simulink model "Dead_Space_Khoo"  (Simulink 6.4)
settings: Solver=ode45  StartTime=0.0  StopTime=10.0  RelTol=1e-3
values from neighbouring files (symbols this model uses):
  Dead1CO2IC = 0.1020    (= 0.102)    [Dead_Space_Khoo_IC.m]    (also in Gas_Exchange_IC.m; Respiratory_IC.m = 39.5616)
  Dead1O2IC = 149.8824    [Dead_Space_Khoo_IC.m]    (also in Gas_Exchange_IC.m; Respiratory_IC.m = 104.3637)
  Dead2CO2IC = 0.5274    [Dead_Space_Khoo_IC.m]    (also in Gas_Exchange_IC.m; Respiratory_IC.m = 39.6736)
  Dead2O2IC = 149.3923    [Dead_Space_Khoo_IC.m]    (also in Gas_Exchange_IC.m; Respiratory_IC.m = 104.2258)
  Dead3CO2IC = 2.2996    [Dead_Space_Khoo_IC.m]    (also in Gas_Exchange_IC.m; Respiratory_IC.m = 39.8127)
  Dead3O2IC = 147.3503    [Dead_Space_Khoo_IC.m]    (also in Gas_Exchange_IC.m; Respiratory_IC.m = 104.0505)
  Dead4CO2IC = 8.2293    [Dead_Space_Khoo_IC.m]    (also in Gas_Exchange_IC.m; Respiratory_IC.m = 40.0061)
  Dead4O2IC = 140.5179    [Dead_Space_Khoo_IC.m]    (also in Gas_Exchange_IC.m; Respiratory_IC.m = 103.8005)
  Dead5CO2IC = 22.0757    [Dead_Space_Khoo_IC.m]    (also in Gas_Exchange_IC.m; Respiratory_IC.m = 40.3359)
  Dead5O2IC = 124.5641    [Dead_Space_Khoo_IC.m]    (also in Gas_Exchange_IC.m; Respiratory_IC.m = 103.3579)
  PICO2 = 0    [Dead_Space_Khoo_IC.m]    (also in Gas_Exchange_IC.m; Respiratory_IC.m)
  PICO2_change = 0    [Respiratory_IC.m]
  PIO2 = 150    [Dead_Space_Khoo_IC.m]    (also in Gas_Exchange_IC.m; Respiratory_IC.m)
  PIO2_change = -90    [Mech_vent_test.m]    (also in Respiratory_IC.m = 0)
  t_CO2_duration = 0    [Respiratory_IC.m]
  t_CO2_start = 0    [Respiratory_IC.m]
  t_O2_duration = 0    [Mech_vent_test.m]    (also in Respiratory_IC.m)
  t_O2_start = 0    [Mech_vent_test.m]    (also in Respiratory_IC.m)
  Vdead1 = 0.03    [Dead_Space_Khoo_IC.m]    (also in Gas_Exchange_IC.m; Respiratory_IC.m)
  Vdead2 = 0.03    [Dead_Space_Khoo_IC.m]    (also in Gas_Exchange_IC.m; Respiratory_IC.m)
  Vdead3 = 0.03    [Dead_Space_Khoo_IC.m]    (also in Gas_Exchange_IC.m; Respiratory_IC.m)
  Vdead4 = 0.03    [Dead_Space_Khoo_IC.m]    (also in Gas_Exchange_IC.m; Respiratory_IC.m)
  Vdead5 = 0.03    [Dead_Space_Khoo_IC.m]    (also in Gas_Exchange_IC.m; Respiratory_IC.m)
settings Model: LastModifiedBy=CLM
settings OptimizationCC: BlockReduction=off  BooleanDataType=off
settings DebuggingCC: SolverPrmCheckMsg=none  StrictBusMsg=None
settings HardwareCC: TargetUnknown=on

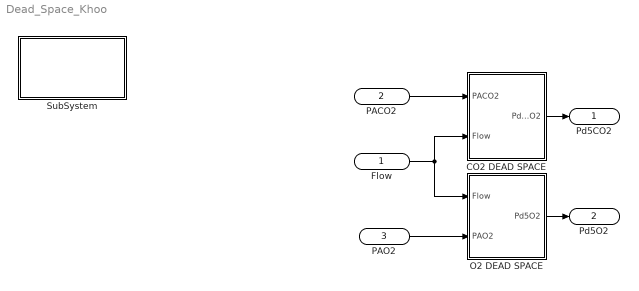
== system Dead_Space_Khoo ==
  Flow : Inport
  PACO2 : Inport  Port=2
  PAO2 : Inport  Port=3
  CO2 DEAD SPACE : Subsystem
  O2 DEAD SPACE : Subsystem
  SubSystem : Subsystem
      settings: OpenFcn=Baro_Ursino_IC
      mask Display: disp('"double click here"\n to load \nDead_Space_Khoo \ninitial values');
  Pd5CO2 : Outport
  Pd5O2 : Outport  Port=2
  wires:
  Flow/1 -> CO2 DEAD SPACE/2(Flow), O2 DEAD SPACE/1(Flow)
  O2 DEAD SPACE/1(Pd5O2) -> Pd5O2/1
  CO2 DEAD SPACE/1(Pd5CO2) -> Pd5CO2/1
  PAO2/1 -> O2 DEAD SPACE/2(PAO2)
  PACO2/1 -> CO2 DEAD SPACE/1(PACO2)

== system Dead_Space_Khoo/CO2 DEAD SPACE ==
  PACO2 : Inport
  Flow : Inport  Port=2
  CO2 Partial Pressure : Subsystem  mask{begin_time=t_CO2_start, end_time=t_CO2_start+t_CO2_duration, init_value=PICO2, final_value=PICO2+PICO2_change}
      mask prompts: begin_time "pulse begin"; end_time "pulse end"; init_value "initial value"; final_value "final value"
      mask Display: disp('pulse')
  Pd(1)CO2 : Subsystem
  Pd(2)CO2 : Subsystem
  Pd(3)CO2 : Subsystem
  Pd(4)CO2 : Subsystem
  Pd(5)CO2 : Subsystem
  Pd5CO2 : Outport
  wires:
  Pd(4)CO2/1(Pd(4)CO2) -> Pd(3)CO2/3(Pd(4)CO2), Pd(5)CO2/1(Pd(4)CO2)
  Pd(3)CO2/1(Pd(3)CO2) -> Pd(2)CO2/3(Pd(3)CO2), Pd(4)CO2/1(Pd(3)CO2)
  Pd(2)CO2/1(Pd(2)CO2) -> Pd(1)CO2/3(Pd(2)CO2), Pd(3)CO2/1(Pd(2)CO2)
  Pd(1)CO2/1(Pd(1)CO2) -> Pd(2)CO2/1(Pd(1)CO2)
  Flow/1 -> Pd(1)CO2/2(Flow), Pd(2)CO2/2(Flow), Pd(5)CO2/2(Flow), Pd(4)CO2/2(Flow), Pd(3)CO2/2(Flow)
  PACO2/1 -> Pd(5)CO2/3(PACO2)
  Pd(5)CO2/1(Pd(5)CO2) -> Pd5CO2/1, Pd(4)CO2/3(Pd(5)CO2)
  CO2 Partial Pressure/1(Out1) -> Pd(1)CO2/1(PICO2)

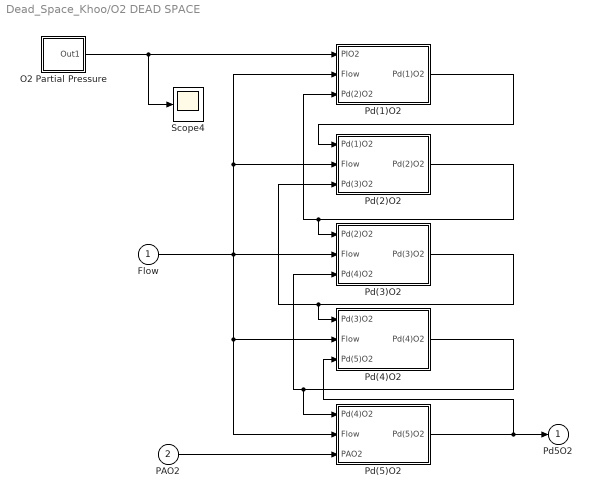
== system Dead_Space_Khoo/O2 DEAD SPACE ==
  Flow : Inport
  PAO2 : Inport  Port=2
  O2 Partial Pressure : Subsystem  mask{begin_time=t_O2_start, end_time=t_O2_start+t_O2_duration, init_value=PIO2, final_value=PIO2+PIO2_change}
      mask prompts: begin_time "pulse begin"; end_time "pulse end"; init_value "initial value"; final_value "final value"
      mask Display: disp('pulse')
  Pd(1)O2 : Subsystem
  Pd(2)O2 : Subsystem
  Pd(3)O2 : Subsystem
  Pd(4)O2 : Subsystem
  Pd(5)O2 : Subsystem
  Scope4 : Scope
      settings: YMin=97.7  YMax=98.3  SaveName=ScopeData40
  Pd5O2 : Outport
  wires:
  Pd(4)O2/1(Pd(4)O2) -> Pd(5)O2/1(Pd(4)O2), Pd(3)O2/3(Pd(4)O2)
  Pd(3)O2/1(Pd(3)O2) -> Pd(2)O2/3(Pd(3)O2), Pd(4)O2/1(Pd(3)O2)
  Pd(2)O2/1(Pd(2)O2) -> Pd(1)O2/3(Pd(2)O2), Pd(3)O2/1(Pd(2)O2)
  Pd(1)O2/1(Pd(1)O2) -> Pd(2)O2/1(Pd(1)O2)
  PAO2/1 -> Pd(5)O2/3(PAO2)
  Flow/1 -> Pd(5)O2/2(Flow), Pd(4)O2/2(Flow), Pd(1)O2/2(Flow), Pd(2)O2/2(Flow), Pd(3)O2/2(Flow)
  Pd(5)O2/1(Pd(5)O2) -> Pd5O2/1, Pd(4)O2/3(Pd(5)O2)
  O2 Partial Pressure/1(Out1) -> Pd(1)O2/1(PIO2), Scope4/1

== system Dead_Space_Khoo/SubSystem ==

== system Dead_Space_Khoo/CO2 DEAD SPACE/CO2 Partial Pressure ==
  Step : Step  Time=begin_time  Before=init_value  After=final_value  SampleTime=0
  Step1 : Step  Time=end_time  After=init_value-final_value  SampleTime=0
  Sum : Sum  Inputs=|++  SaturateOnIntegerOverflow=on  InputSameDT=on
  Out1 : Outport
  wires:
  Step/1 -> Sum/1
  Step1/1 -> Sum/2
  Sum/1 -> Out1/1

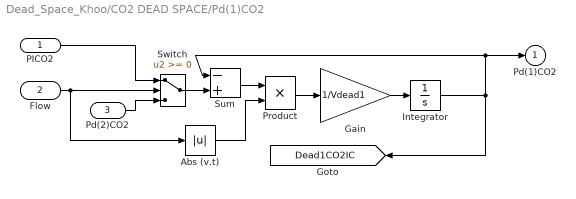
== system Dead_Space_Khoo/CO2 DEAD SPACE/Pd(1)CO2 ==
  PICO2 : Inport
  Flow : Inport  Port=2
  Pd(2)CO2 : Inport  Port=3
  Abs (v.t) : Abs  SaturateOnIntegerOverflow=on  SampleTime=-1
  Gain : Gain  Gain=1/Vdead1  SaturateOnIntegerOverflow=on
  Integrator : Integrator  InitialCondition=Dead1CO2IC
  Product : Product  SaturateOnIntegerOverflow=on  RndMeth=Zero  InputSameDT=on
  Sum : Sum  Inputs=-+  SaturateOnIntegerOverflow=on  InputSameDT=on
  Switch : Switch  SaturateOnIntegerOverflow=on  InputSameDT=on
  Pd(1)CO2 : Outport
  tag scope: Dead1CO2IC=global
  wires:
  Flow/1 -> Abs (v.t)/1, Switch/2
  Abs (v.t)/1 -> Product/2
  Switch/1 -> Sum/2
  Product/1 -> Gain/1
  Gain/1 -> Integrator/1
  Integrator/1 -> Sum/1, Pd(1)CO2/1, [Dead1CO2IC]
  Sum/1 -> Product/1
  PICO2/1 -> Switch/1
  Pd(2)CO2/1 -> Switch/3

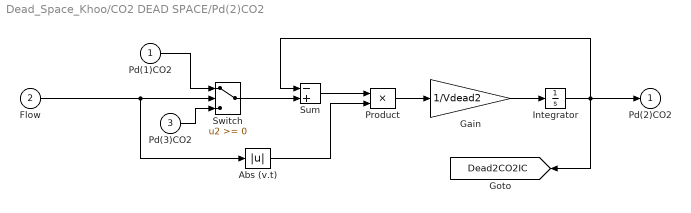
== system Dead_Space_Khoo/CO2 DEAD SPACE/Pd(2)CO2 ==
  Pd(1)CO2 : Inport
  Flow : Inport  Port=2
  Pd(3)CO2 : Inport  Port=3
  Abs (v.t) : Abs  SaturateOnIntegerOverflow=on  SampleTime=-1
  Gain : Gain  Gain=1/Vdead2  SaturateOnIntegerOverflow=on
  Integrator : Integrator  InitialCondition=Dead2CO2IC
  Product : Product  SaturateOnIntegerOverflow=on  RndMeth=Zero  InputSameDT=on
  Sum : Sum  Inputs=-+  SaturateOnIntegerOverflow=on  InputSameDT=on
  Switch : Switch  SaturateOnIntegerOverflow=on  InputSameDT=on
  Pd(2)CO2 : Outport
  tag scope: Dead2CO2IC=global
  wires:
  Integrator/1 -> Sum/1, Pd(2)CO2/1, [Dead2CO2IC]
  Abs (v.t)/1 -> Product/2
  Flow/1 -> Abs (v.t)/1, Switch/2
  Pd(3)CO2/1 -> Switch/3
  Pd(1)CO2/1 -> Switch/1
  Sum/1 -> Product/1
  Gain/1 -> Integrator/1
  Product/1 -> Gain/1
  Switch/1 -> Sum/2

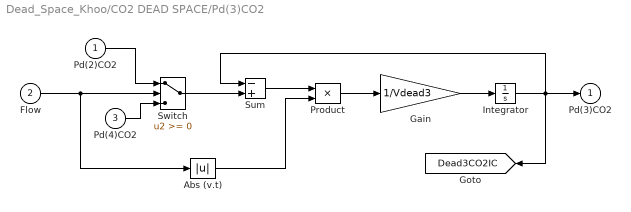
== system Dead_Space_Khoo/CO2 DEAD SPACE/Pd(3)CO2 ==
  Pd(2)CO2 : Inport
  Flow : Inport  Port=2
  Pd(4)CO2 : Inport  Port=3
  Abs (v.t) : Abs  SaturateOnIntegerOverflow=on  SampleTime=-1
  Gain : Gain  Gain=1/Vdead3  SaturateOnIntegerOverflow=on
  Integrator : Integrator  InitialCondition=Dead3CO2IC
  Product : Product  SaturateOnIntegerOverflow=on  RndMeth=Zero  InputSameDT=on
  Sum : Sum  Inputs=-+  SaturateOnIntegerOverflow=on  InputSameDT=on
  Switch : Switch  SaturateOnIntegerOverflow=on  InputSameDT=on
  Pd(3)CO2 : Outport
  tag scope: Dead3CO2IC=global
  wires:
  Abs (v.t)/1 -> Product/2
  Flow/1 -> Abs (v.t)/1, Switch/2
  Switch/1 -> Sum/2
  Product/1 -> Gain/1
  Gain/1 -> Integrator/1
  Integrator/1 -> Sum/1, Pd(3)CO2/1, [Dead3CO2IC]
  Sum/1 -> Product/1
  Pd(2)CO2/1 -> Switch/1
  Pd(4)CO2/1 -> Switch/3

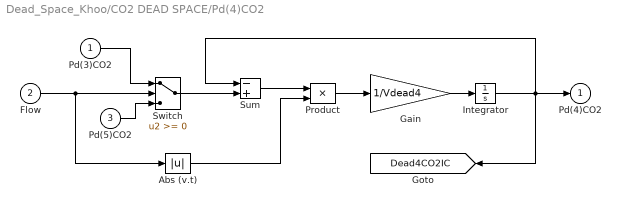
== system Dead_Space_Khoo/CO2 DEAD SPACE/Pd(4)CO2 ==
  Pd(3)CO2 : Inport
  Flow : Inport  Port=2
  Pd(5)CO2 : Inport  Port=3
  Abs (v.t) : Abs  SaturateOnIntegerOverflow=on  SampleTime=-1
  Gain : Gain  Gain=1/Vdead4  SaturateOnIntegerOverflow=on
  Integrator : Integrator  InitialCondition=Dead4CO2IC
  Product : Product  SaturateOnIntegerOverflow=on  RndMeth=Zero  InputSameDT=on
  Sum : Sum  Inputs=-+  SaturateOnIntegerOverflow=on  InputSameDT=on
  Switch : Switch  SaturateOnIntegerOverflow=on  InputSameDT=on
  Pd(4)CO2 : Outport
  tag scope: Dead4CO2IC=global
  wires:
  Integrator/1 -> Sum/1, Pd(4)CO2/1, [Dead4CO2IC]
  Abs (v.t)/1 -> Product/2
  Flow/1 -> Abs (v.t)/1, Switch/2
  Pd(5)CO2/1 -> Switch/3
  Pd(3)CO2/1 -> Switch/1
  Sum/1 -> Product/1
  Gain/1 -> Integrator/1
  Product/1 -> Gain/1
  Switch/1 -> Sum/2

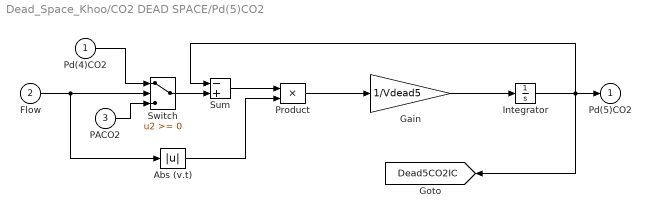
== system Dead_Space_Khoo/CO2 DEAD SPACE/Pd(5)CO2 ==
  Pd(4)CO2 : Inport
  Flow : Inport  Port=2
  PACO2 : Inport  Port=3
  Abs (v.t) : Abs  SaturateOnIntegerOverflow=on  SampleTime=-1
  Gain : Gain  Gain=1/Vdead5  SaturateOnIntegerOverflow=on
  Integrator : Integrator  InitialCondition=Dead5CO2IC
  Product : Product  SaturateOnIntegerOverflow=on  RndMeth=Zero  InputSameDT=on
  Sum : Sum  Inputs=-+  SaturateOnIntegerOverflow=on  InputSameDT=on
  Switch : Switch  SaturateOnIntegerOverflow=on  InputSameDT=on
  Pd(5)CO2 : Outport
  tag scope: Dead5CO2IC=global
  wires:
  Abs (v.t)/1 -> Product/2
  Flow/1 -> Abs (v.t)/1, Switch/2
  Switch/1 -> Sum/2
  Product/1 -> Gain/1
  Gain/1 -> Integrator/1
  Integrator/1 -> Sum/1, Pd(5)CO2/1, [Dead5CO2IC]
  Sum/1 -> Product/1
  Pd(4)CO2/1 -> Switch/1
  PACO2/1 -> Switch/3

== system Dead_Space_Khoo/O2 DEAD SPACE/O2 Partial Pressure ==
  Step : Step  Time=begin_time  Before=init_value  After=final_value  SampleTime=0
  Step1 : Step  Time=end_time  After=init_value-final_value  SampleTime=0
  Sum : Sum  Inputs=|++  SaturateOnIntegerOverflow=on  InputSameDT=on
  Out1 : Outport
  wires:
  Sum/1 -> Out1/1
  Step1/1 -> Sum/2
  Step/1 -> Sum/1

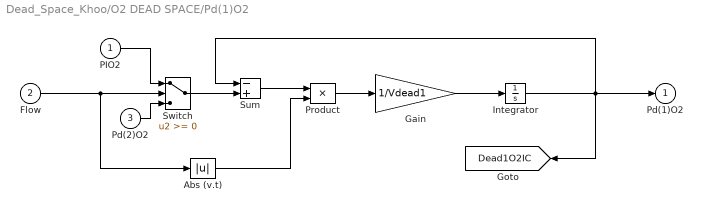
== system Dead_Space_Khoo/O2 DEAD SPACE/Pd(1)O2 ==
  PIO2 : Inport
  Flow : Inport  Port=2
  Pd(2)O2 : Inport  Port=3
  Abs (v.t) : Abs  SaturateOnIntegerOverflow=on  SampleTime=-1
  Gain : Gain  Gain=1/Vdead1  SaturateOnIntegerOverflow=on
  Integrator : Integrator  InitialCondition=Dead1O2IC
  Product : Product  SaturateOnIntegerOverflow=on  RndMeth=Zero  InputSameDT=on
  Sum : Sum  Inputs=-+  SaturateOnIntegerOverflow=on  InputSameDT=on
  Switch : Switch  SaturateOnIntegerOverflow=on  InputSameDT=on
  Pd(1)O2 : Outport
  tag scope: Dead1O2IC=global
  wires:
  Switch/1 -> Sum/2
  Pd(2)O2/1 -> Switch/3
  PIO2/1 -> Switch/1
  Sum/1 -> Product/1
  Integrator/1 -> Sum/1, Pd(1)O2/1, [Dead1O2IC]
  Gain/1 -> Integrator/1
  Product/1 -> Gain/1
  Flow/1 -> Abs (v.t)/1, Switch/2
  Abs (v.t)/1 -> Product/2

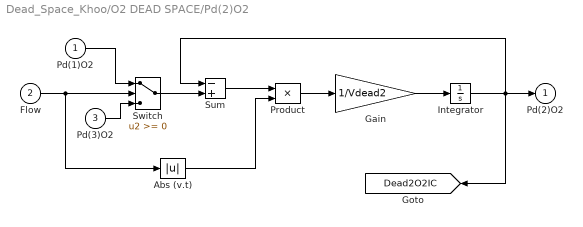
== system Dead_Space_Khoo/O2 DEAD SPACE/Pd(2)O2 ==
  Pd(1)O2 : Inport
  Flow : Inport  Port=2
  Pd(3)O2 : Inport  Port=3
  Abs (v.t) : Abs  SaturateOnIntegerOverflow=on  SampleTime=-1
  Gain : Gain  Gain=1/Vdead2  SaturateOnIntegerOverflow=on
  Integrator : Integrator  InitialCondition=Dead2O2IC
  Product : Product  SaturateOnIntegerOverflow=on  RndMeth=Zero  InputSameDT=on
  Sum : Sum  Inputs=-+  SaturateOnIntegerOverflow=on  InputSameDT=on
  Switch : Switch  SaturateOnIntegerOverflow=on  InputSameDT=on
  Pd(2)O2 : Outport
  tag scope: Dead2O2IC=global
  wires:
  Abs (v.t)/1 -> Product/2
  Flow/1 -> Abs (v.t)/1, Switch/2
  Product/1 -> Gain/1
  Integrator/1 -> [Dead2O2IC], Sum/1, Pd(2)O2/1
  Sum/1 -> Product/1
  Pd(1)O2/1 -> Switch/1
  Pd(3)O2/1 -> Switch/3
  Switch/1 -> Sum/2
  Gain/1 -> Integrator/1

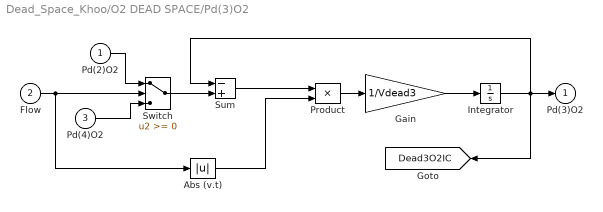
== system Dead_Space_Khoo/O2 DEAD SPACE/Pd(3)O2 ==
  Pd(2)O2 : Inport
  Flow : Inport  Port=2
  Pd(4)O2 : Inport  Port=3
  Abs (v.t) : Abs  SaturateOnIntegerOverflow=on  SampleTime=-1
  Gain : Gain  Gain=1/Vdead3  SaturateOnIntegerOverflow=on
  Integrator : Integrator  InitialCondition=Dead3O2IC
  Product : Product  SaturateOnIntegerOverflow=on  RndMeth=Zero  InputSameDT=on
  Sum : Sum  Inputs=-+  SaturateOnIntegerOverflow=on  InputSameDT=on
  Switch : Switch  SaturateOnIntegerOverflow=on  InputSameDT=on
  Pd(3)O2 : Outport
  tag scope: Dead3O2IC=global
  wires:
  Switch/1 -> Sum/2
  Pd(4)O2/1 -> Switch/3
  Pd(2)O2/1 -> Switch/1
  Sum/1 -> Product/1
  Integrator/1 -> [Dead3O2IC], Sum/1, Pd(3)O2/1
  Product/1 -> Gain/1
  Flow/1 -> Abs (v.t)/1, Switch/2
  Abs (v.t)/1 -> Product/2
  Gain/1 -> Integrator/1

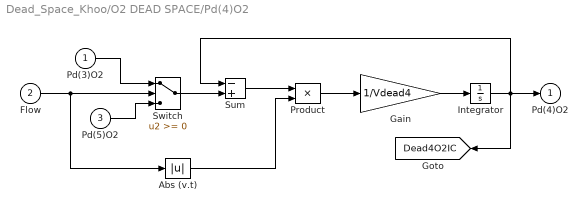
== system Dead_Space_Khoo/O2 DEAD SPACE/Pd(4)O2 ==
  Pd(3)O2 : Inport
  Flow : Inport  Port=2
  Pd(5)O2 : Inport  Port=3
  Abs (v.t) : Abs  SaturateOnIntegerOverflow=on  SampleTime=-1
  Gain : Gain  Gain=1/Vdead4  SaturateOnIntegerOverflow=on
  Integrator : Integrator  InitialCondition=Dead4O2IC
  Product : Product  SaturateOnIntegerOverflow=on  RndMeth=Zero  InputSameDT=on
  Sum : Sum  Inputs=-+  SaturateOnIntegerOverflow=on  InputSameDT=on
  Switch : Switch  SaturateOnIntegerOverflow=on  InputSameDT=on
  Pd(4)O2 : Outport
  tag scope: Dead4O2IC=global
  wires:
  Abs (v.t)/1 -> Product/2
  Flow/1 -> Abs (v.t)/1, Switch/2
  Product/1 -> Gain/1
  Integrator/1 -> Sum/1, Pd(4)O2/1, [Dead4O2IC]
  Sum/1 -> Product/1
  Pd(3)O2/1 -> Switch/1
  Pd(5)O2/1 -> Switch/3
  Switch/1 -> Sum/2
  Gain/1 -> Integrator/1

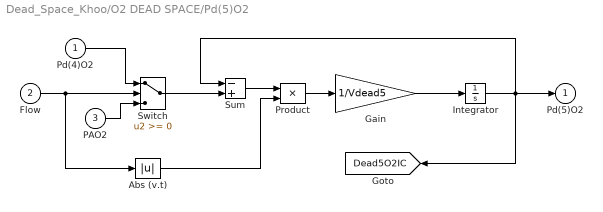
== system Dead_Space_Khoo/O2 DEAD SPACE/Pd(5)O2 ==
  Pd(4)O2 : Inport
  Flow : Inport  Port=2
  PAO2 : Inport  Port=3
  Abs (v.t) : Abs  SaturateOnIntegerOverflow=on  SampleTime=-1
  Gain : Gain  Gain=1/Vdead5  SaturateOnIntegerOverflow=on
  Integrator : Integrator  InitialCondition=Dead5O2IC
  Product : Product  SaturateOnIntegerOverflow=on  RndMeth=Zero  InputSameDT=on
  Sum : Sum  Inputs=-+  SaturateOnIntegerOverflow=on  InputSameDT=on
  Switch : Switch  SaturateOnIntegerOverflow=on  InputSameDT=on
  Pd(5)O2 : Outport
  tag scope: Dead5O2IC=global
  wires:
  Switch/1 -> Sum/2
  PAO2/1 -> Switch/3
  Pd(4)O2/1 -> Switch/1
  Sum/1 -> Product/1
  Integrator/1 -> Sum/1, Pd(5)O2/1, [Dead5O2IC]
  Product/1 -> Gain/1
  Flow/1 -> Abs (v.t)/1, Switch/2
  Abs (v.t)/1 -> Product/2
  Gain/1 -> Integrator/1
